simulink model "Copy_of_Subsystem"  (R2020b)
settings: Solver=FixedStepAuto  StartTime=0.0  StopTime=10.0  FixedStep=0.1  RelTol=1e-3
settings Model: Creator=Lenovo  LastModifiedBy=Lenovo
settings DataIOCC: SaveOutput=off  SaveTime=off

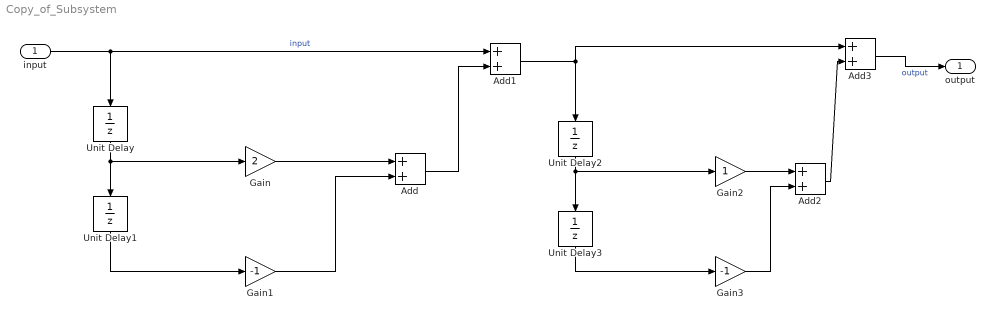
== system Copy_of_Subsystem ==
  input : Inport  OutDataTypeStr=double  PortDimensions=1  SampleTime=[0.10000000000000001,0]
  Add{,1..3} (4 alike) : Sum
  Gain : Gain  Gain=2
  Gain1 : Gain  Gain=-1
  Gain2 : Gain
  Gain3 : Gain  Gain=-1
  Unit Delay{,1..3} (4 alike) : UnitDelay  SampleTime=-1  HasFrameUpgradeWarning=on
  output : Outport  OutDataTypeStr=double  PortDimensions=1  SampleTime=[0.10000000000000001,0]
  wires:
  Add1/1 -> Add3/1, Unit Delay2/1
  Gain3/1 -> Add2/2
  input/1 -> Add1/1, Unit Delay/1  "input"
  Unit Delay/1 -> Unit Delay1/1, Gain/1
  Gain2/1 -> Add2/1
  Unit Delay2/1 -> Unit Delay3/1, Gain2/1
  Gain1/1 -> Add/2
  Add2/1 -> Add3/2
  Gain/1 -> Add/1
  Add/1 -> Add1/2
  Unit Delay1/1 -> Gain1/1
  Add3/1 -> output/1  "output"
  Unit Delay3/1 -> Gain3/1
